simulink model "Cube"  (R2023a)
settings: Solver=FixedStepAuto  StartTime=0.0  StopTime=5  FixedStep=0.001  RelTol=1e-3
settings Model: Creator=Joseph Maher Labib  LastModifiedBy=totae
settings OptimizationCC: DefaultParameterBehavior=Inlined  EnhancedBackFolding=on  PassReuseOutputArgsAs=Individual arguments  ZeroExternalMemoryAtStartup=off  ZeroInternalMemoryAtStartup=off  OptimizeBlockOrder=speed  DifferentSizesBufferReuse=on  OptimizationCustomize=off  EfficientTunableParamExpr=on
settings DebuggingCC: ParameterTunabilityLossMsg=error
settings SFSimCC: MATLABDynamicMemAlloc=off
settings RTWCC: Description=Create Visual C/C++ Solution File for Embedded Coder  SystemTargetFile=ert.tlc  TemplateMakefile=RTW.MSVCBuild
settings CodeAppCC: ForceParamTrailComments=on  IgnoreCustomStorageClasses=off  OperatorAnnotations=on  SimulinkDataObjDesc=on  SFDataObjDesc=on  InsertBlockDesc=on
settings ERTTargetCC: TargetLangStandard=C99 (ISO)  GenerateSampleERTMain=on  SupportContinuousTime=on  InlinedParameterPlacement=NonHierarchical  ERTCustomFileTemplate=example_file_process.tlc

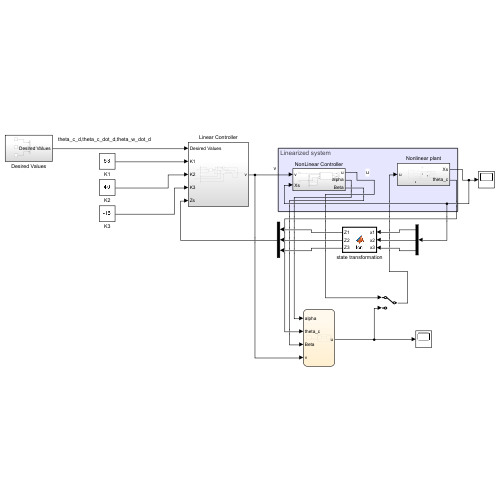
[thumbnail: Simulink's stored preview of the top-level diagram]
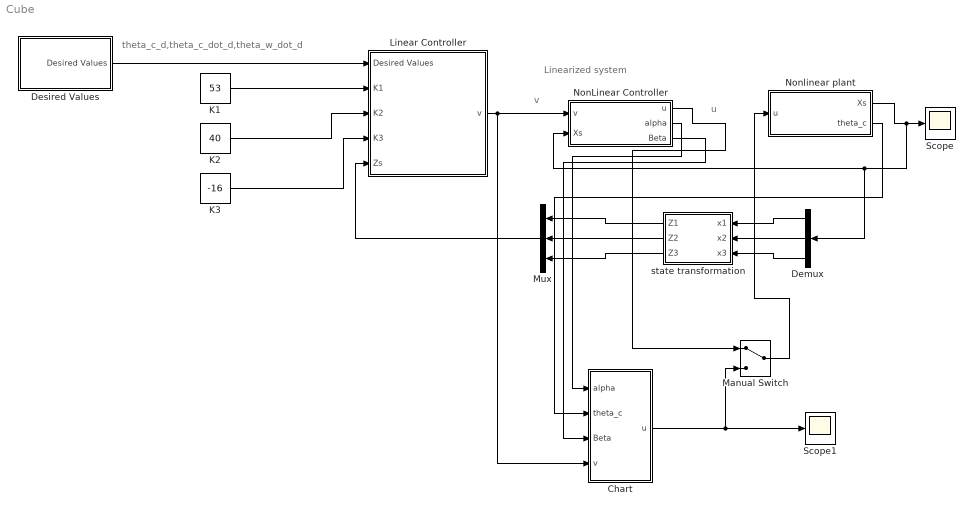
== system Cube ==
  note: Linearized system
  note: u
  note: v
  note: theta_c_d,theta_c_dot_d,theta_w_dot_d
  Chart : Stateflow chart  TreatAsAtomicUnit=on
  Demux : Demux  Outputs=3
  Desired Values : Subsystem
  K1 : Constant  Value=53
  K2 : Constant  Value=40
  K3 : Constant  Value=-16
  Linear Controller : Subsystem
  Manual Switch : ManualSwitch
  Mux : Mux  Inputs=3
  NonLinear Controller : Subsystem
  Nonlinear plant : Subsystem
  Scope : Scope
  Scope1 : Scope
  state transformation : MATLAB Function  TreatAsAtomicUnit=on
  wires:
  Desired Values/1(Desired Values) -> Linear Controller/1(Desired Values)
  Linear Controller/1(v) -> Chart/4(v), NonLinear Controller/1(v)
  NonLinear Controller/1(u) -> Manual Switch/1
  K1/1 -> Linear Controller/2(K1)
  K2/1 -> Linear Controller/3(K2)
  K3/1 -> Linear Controller/4(K3)
  Nonlinear plant/1(Xs) -> Demux/1, NonLinear Controller/2(Xs), Scope/1
  Demux/1 -> state transformation/1(x1)
  Demux/2 -> state transformation/2(x2)
  Demux/3 -> state transformation/3(x3)
  state transformation/2(Z2) -> Mux/2
  state transformation/1(Z1) -> Mux/1
  state transformation/3(Z3) -> Mux/3
  Mux/1 -> Linear Controller/5(Zs)
  NonLinear Controller/2(alpha) -> Chart/1(alpha)
  NonLinear Controller/3(Beta) -> Chart/3(Beta)
  Nonlinear plant/2(theta_c) -> Chart/2(theta_c)
  Chart/1(u) -> Manual Switch/2, Scope1/1
  Manual Switch/1 -> Nonlinear plant/1(u)

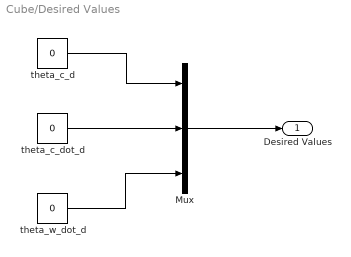
== system Cube/Desired Values ==
  Mux : Mux  Inputs=3
  theta_c_d : Constant  Value=0
  theta_c_dot_d : Constant  Value=0
  theta_w_dot_d : Constant  Value=0
  Desired Values : Outport
  wires:
  theta_c_dot_d/1 -> Mux/2
  theta_c_d/1 -> Mux/1
  theta_w_dot_d/1 -> Mux/3
  Mux/1 -> Desired Values/1

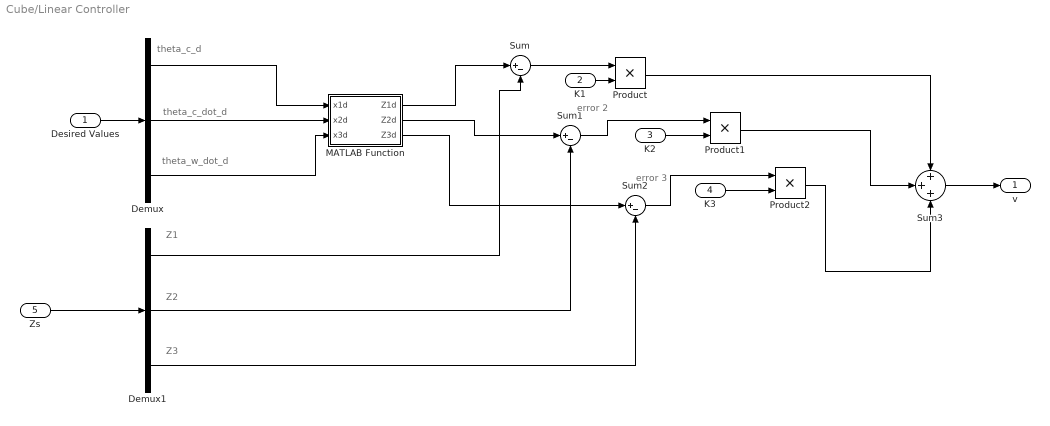
== system Cube/Linear Controller ==
  note: error 2
  note: error 3
  note: theta_w_dot_d
  note: theta_c_dot_d
  note: theta_c_d
  note: Z1
  note: Z2
  note: Z3
  Desired Values : Inport
  K1 : Inport  Port=2
  K2 : Inport  Port=3
  K3 : Inport  Port=4
  Zs : Inport  Port=5
  Demux : Demux  Outputs=3
  Demux1 : Demux  Outputs=3
  MATLAB Function : MATLAB Function  TreatAsAtomicUnit=on
  Product : Product
  Product1 : Product
  Product2 : Product
  Sum : Sum  Inputs=|+-
  Sum1 : Sum  Inputs=|+-
  Sum2 : Sum  Inputs=|+-
  Sum3 : Sum  Inputs=+++
  v : Outport
  wires:
  Desired Values/1 -> Demux/1
  Zs/1 -> Demux1/1
  Demux1/1 -> Sum/2
  Demux1/2 -> Sum1/2
  Demux1/3 -> Sum2/2
  K1/1 -> Product/2
  K2/1 -> Product1/2
  K3/1 -> Product2/2
  Product/1 -> Sum3/1
  Product1/1 -> Sum3/2
  Product2/1 -> Sum3/3
  Sum3/1 -> v/1
  Demux/1 -> MATLAB Function/1(x1d)
  Demux/2 -> MATLAB Function/2(x2d)
  Demux/3 -> MATLAB Function/3(x3d)
  MATLAB Function/1(Z1d) -> Sum/1
  MATLAB Function/3(Z3d) -> Sum2/1
  Sum2/1 -> Product2/1
  MATLAB Function/2(Z2d) -> Sum1/1
  Sum1/1 -> Product1/1
  Sum/1 -> Product/1

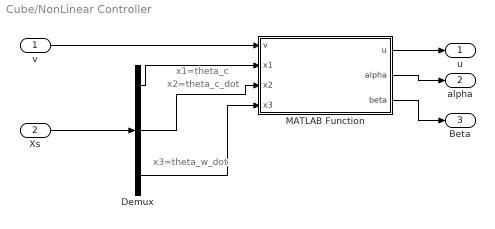
== system Cube/NonLinear Controller ==
  note: x1=theta_c
  note: x2=theta_c_dot
  note: x3=theta_w_dot
  v : Inport
  Xs : Inport  Port=2
  Demux : Demux  Outputs=3
  MATLAB Function : MATLAB Function  TreatAsAtomicUnit=on
  u : Outport
  alpha : Outport  Port=2
  Beta : Outport  Port=3
  wires:
  Xs/1 -> Demux/1
  v/1 -> MATLAB Function/1(v)
  Demux/1 -> MATLAB Function/2(x1)
  Demux/2 -> MATLAB Function/3(x2)
  Demux/3 -> MATLAB Function/4(x3)
  MATLAB Function/1(u) -> u/1
  MATLAB Function/2(alpha) -> alpha/1
  MATLAB Function/3(beta) -> Beta/1

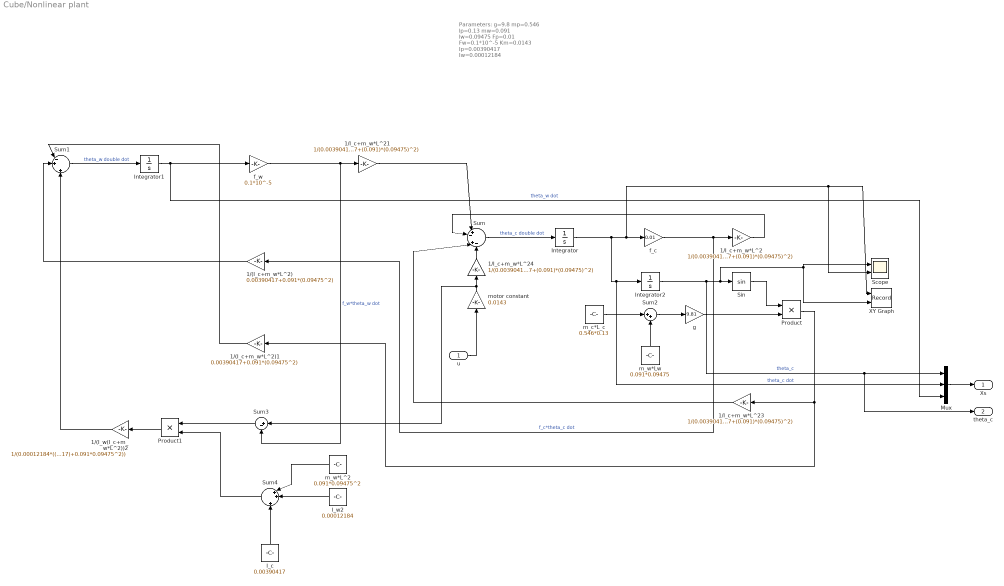
== system Cube/Nonlinear plant ==
  note: Parameters:
      | g=9.8
      | mp=0.546
      | lp=0.13
      | mw=0.091
      | lw=0.09475
      | Fp=0.01
      | Fw=0.1*10^-5
      | Km=0.0143
      | Ip=0.00390417
      | Iw=0.00012184
  u : Inport
  1/(I_c+m_w*L^2) : Gain  Gain=0.00390417+0.091*(0.09475^2)
  1/(I_c+m_w*L^2)1 : Gain  Gain=0.00390417+0.091*(0.09475^2)
  1/(I_w(I_c+m_w*L^2))2 : Gain  Gain=1/(0.00012184*((0.00390417)+0.091*0.09475^2))
  1/I_c+m_w*L^{2,21,23..24} (4 alike) : Gain  Gain=1/(0.00390417+(0.091)*(0.09475)^2)
  I_c : Constant  Value=0.00390417
  I_w2 : Constant  Value=0.00012184
  Integrator : Integrator
  Integrator1 : Integrator
  Integrator2 : Integrator
  Mux : Mux  Inputs=3
  Product : Product
  Product1 : Product
  Scope : Scope  NumInputPorts=2
  Sin : Trigonometry
  Sum : Sum  Inputs=|+-|+-
  Sum1 : Sum  Inputs=|-+|+
  Sum2 : Sum  Inputs=|++
  Sum3 : Sum  Inputs=|+-
  Sum4 : Sum  Inputs=|++|+
  XY Graph : Record  FileSettingsInternal="{\"entries\":[{\"content\":{\"excelSettings\":{\"content\":{},\"type\":\"Streamout.ExcelSettings\"}},\"type\":\"Streamout.FileSettingStorage\",\"uuid\":\"66a67cd6-09ae-4402-aca9-595720089f73\"}],\"packageUris\":[\"http://schema.mathworks.com/mf0/streamout_blocks/R2020a\"],\"version\":\"1.0\"}"  Layout=[1 1]  SignalsInternal="{\"entries\":[{\"content\":{\"signals\":[{\"content\":{\"blockPath\":[\"Cube/Nonlinear plant/XY Graph\"],\"dimensions\":[1],\"domain\":\"Cube/Nonlinear plant/XY Graph\",\"lineColor\":\"#0072bd\",\"plots\":[1],\"port\":1,\"signalID\":780,\"signalName\":\"theta_c dot\"},\"type\":\"RecordBlkView.Signal\",\"uuid\":\"a54ead99-843e-44f8-bb7c-9abc90be0651\"},{\"content\":{\"blockPath\":[\"Cube/Nonlinear plant/XY Graph\"],\"dimensions\":[1],\"domain\":\"Cube/Nonlinear plant/XY Graph\",\"lineColor\":\"#d95319\",\"plots\":[1],\"port\":2,\"signalID\":783,\"signalName\":\"theta_c\"},\"type\":\"RecordBlkView.Signal\",\"uuid\":\"b884fb43-d68a-49de-818e-e16d103745a3\"}]},\"type\":\"RecordBlkView.InputSignals\",\"uuid\":\"03c16a7e-bf53-4f70-b834-54f942da8cff\"}],\"packageUris\":[\"http://schema.mathworks.com/mf0/streamout_blocks/R2020a\"],\"version\":\"1.0\"}"  VisualizationBindings="{\"xyplotplugin\":{\"info\":[{\"series\":[{\"bindingParametersList\":[{\"parameter\":\"Y-Axis\",\"signalID\":780,\"signalName\":\"theta_c dot\"},{\"parameter\":\"X-Axis\",\"signalID\":783,\"signalName\":\"theta_c\"}],\"seriesID\":4721}],\"subplotID\":1}]}}"  CompatibilityTag=XY
  f_c : Gain  Gain=0.01
  f_w : Gain  Gain=0.1*10^-5
  g : Gain  Gain=9.81
  m_c*L_c : Constant  Value=0.546*0.13
  m_w*L^2 : Constant  Value=0.091*0.09475^2
  m_w*Lw : Constant  Value=0.091*0.09475
  motor constant : Gain  Gain=0.0143
  Xs : Outport
  theta_c : Outport  Port=2
  wires:
  I_w2/1 -> Sum4/2
  Integrator/1 -> Mux/2, Integrator2/1, XY Graph/1, Scope/2, f_c/1  "theta_c dot"
  Sin/1 -> Product/1
  I_c/1 -> Sum4/3
  Sum3/1 -> Product1/1
  1/I_c+m_w*L^21/1 -> Sum/1
  1/(I_w(I_c+m_w*L^2))2/1 -> Sum1/3
  Product1/1 -> 1/(I_w(I_c+m_w*L^2))2/1
  m_w*L^2/1 -> Sum4/1
  Integrator1/1 -> Mux/3, f_w/1  "theta_w dot"
  1/I_c+m_w*L^24/1 -> Sum/4
  m_w*Lw/1 -> Sum2/2
  1/(I_c+m_w*L^2)/1 -> Sum1/2
  Product/1 -> 1/(I_c+m_w*L^2)1/1, 1/I_c+m_w*L^23/1
  motor constant/1 -> Sum3/1, 1/I_c+m_w*L^24/1
  1/I_c+m_w*L^23/1 -> Sum/3
  Integrator2/1 -> theta_c/1, Mux/1, XY Graph/2, Scope/1, Sin/1  "theta_c"
  Sum4/1 -> Product1/2
  m_c*L_c/1 -> Sum2/1
  u/1 -> motor constant/1
  1/I_c+m_w*L^2/1 -> Sum/2
  Sum/1 -> Integrator/1  "theta_c double dot"
  f_w/1 -> 1/I_c+m_w*L^21/1, Sum3/2  "f_w*theta_w dot"
  f_c/1 -> 1/(I_c+m_w*L^2)/1, 1/I_c+m_w*L^2/1  "f_c*theta_c dot"
  g/1 -> Product/2
  Sum2/1 -> g/1
  Sum1/1 -> Integrator1/1  "theta_w double dot"
  1/(I_c+m_w*L^2)1/1 -> Sum1/1
  Mux/1 -> Xs/1

== stateflow chart Cube/Chart ==
  state On
    state Balanced
      entry:
      during:
      u=0;
    state Falling
      entry:
      during:
      u=alpha+Beta*v;
    (default) -> Balanced
    Balanced -> Falling : [theta_c >5 || theta_c<-5]
    Falling -> Balanced : [theta_c>-5 && theta_c<5]
  state Off
    entry:
    during:
    u=0;
  (default) -> Off
  On -> Off : [button_pressed==0]
  Off -> On : [button_pressed==1]
  data: alpha input; theta_c input; Beta input; v input; u output double; button_pressed local double

== matlab function Cube/NonLinear Controller/MATLAB Function ==
  data: v input; u output; x1 input; x2 input; x3 input; alpha output; beta output
function [u,alpha,beta] = fcn(v,x1,x2,x3)

%Parameters: 
g=9.8;
mp=0.546;
lp=0.13;
mw=0.091;
lw=0.09475;
Fp=0.01;
Fw=0.1*10^-5;
Km=0.0143;
Ip=0.00390417;
Iw=0.00012184;

alpha =(x2*((49*g*x2*sin(x1)*(lp*mp + lw*mw))/(60*(mw*lw^2 + Ip)) - (g*cos(x1)*((11*Fw)/(60*(mw*lw^2 + Ip)) - Fw/(Iw*(mw*lw^2 + Ip)))*(lp*mp + lw*mw))/(mw*lw^2 + Ip) + (g*cos(x1)*((49*Fp)/(60*(mw*lw^2 + Ip)) - 467/225)*(lp*mp + lw*mw))/(mw*lw^2 + Ip)) + ((Fp*x2 - g*sin(x1)*(lp*mp + lw*mw))/(mw*lw^2 + Ip) + (mw*lw^2 + Ip + Iw - Fw*x3)/(Iw*(mw*lw^2 + Ip)))*((Fw*((49*Fp)/(60*(mw*lw^2 + Ip)) - 467/225))/(mw*lw^2 + Ip) - (Fw*((11*Fw)/(60*(mw*lw^2 + Ip)) - Fw/(Iw*(mw*lw^2 + Ip))))/(Iw*(mw*lw^2 + Ip))) - ((Fw*x3 - Fp*x2 + g*sin(x1)*(lp*mp + lw*mw))*((Fp*((49*Fp)/(60*(mw*lw^2 + Ip)) - 467/225))/(mw*lw^2 + Ip) - (Fp*((11*Fw)/(60*(mw*lw^2 + Ip)) - Fw/(Iw*(mw*lw^2 + Ip))))/(mw*lw^2 + Ip) + (49*g*cos(x1)*(lp*mp + lw*mw))/(60*(mw*lw^2 + Ip))))/(mw*lw^2 + Ip))/((Km*((Fp*((49*Fp)/(60*(mw*lw^2 + Ip)) - 467/225))/(mw*lw^2 + Ip) - (Fp*((11*Fw)/(60*(mw*lw^2 + Ip)) - Fw/(Iw*(mw*lw^2 + Ip))))/(mw*lw^2 + Ip) + (49*g*cos(x1)*(lp*mp + lw*mw))/(60*(mw*lw^2 + Ip))))/(mw*lw^2 + Ip) + (Km*(mw*lw^2 + Ip)*((Fw*((49*Fp)/(60*(mw*lw^2 + Ip)) - 467/225))/(mw*lw^2 + Ip) - (Fw*((11*Fw)/(60*(mw*lw^2 + Ip)) - Fw/(Iw*(mw*lw^2 + Ip))))/(Iw*(mw*lw^2 + Ip))))/Iw);
 
beta =1/((Km*((Fp*((49*Fp)/(60*(mw*lw^2 + Ip)) - 467/225))/(mw*lw^2 + Ip) - (Fp*((11*Fw)/(60*(mw*lw^2 + Ip)) - Fw/(Iw*(mw*lw^2 + Ip))))/(mw*lw^2 + Ip) + (49*g*cos(x1)*(lp*mp + lw*mw))/(60*(mw*lw^2 + Ip))))/(mw*lw^2 + Ip) + (Km*(mw*lw^2 + Ip)*((Fw*((49*Fp)/(60*(mw*lw^2 + Ip)) - 467/225))/(mw*lw^2 + Ip) - (Fw*((11*Fw)/(60*(mw*lw^2 + Ip)) - Fw/(Iw*(mw*lw^2 + Ip))))/(Iw*(mw*lw^2 + Ip))))/Iw);


u=alpha+beta*v

== matlab function Cube/state transformation ==
  data: x1 input; Z1 output; x2 input; x3 input; Z2 output; Z3 output
function [Z1,Z2,Z3] = fcn(x1,x2,x3)

%Parameters 
g=9.8;
mp=0.546;
lp=0.13;
mw=0.091;
lw=0.09475;
Fp=0.01;
Fw=0.1*10^-5;
Km=0.0143;
Ip=0.00390417;
Iw=0.00012184;


Z1 = (-467/225)*x1+(11/60)*x2+x3;
Z2 =(Fp*x2 - g*sin(x1)*(lp*mp + lw*mw))/(mw*lw^2 + Ip) - (467*x2)/225 + (11*(Fw*x3 - Fp*x2+ g*sin(x1)*(lp*mp + lw*mw)))/(60*(mw*lw^2 + Ip)) + (mw*lw^2 + Ip + Iw - Fw*x3)/(Iw*(mw*lw^2 + Ip));
Z3 =((11*Fw)/(60*(mw*lw^2 + Ip)) - Fw/(Iw*(mw*lw^2 + Ip)))*((Fp*x2 - g*sin(x1)*(lp*mp + lw*mw))/(mw*lw^2 + Ip) + (mw*lw^2 + Ip + Iw - Fw*x3)/(Iw*(mw*lw^2 + Ip))) + (((49*Fp)/(60*(mw*lw^2 + Ip)) - 467/225)*(Fw*x3 - Fp*x2 + g*sin(x1)*(lp*mp + lw*mw)))/(mw*lw^2 + Ip) - (49*g*x2*cos(x1)*(lp*mp + lw*mw))/(60*(mw*lw^2 + Ip));

== matlab function Cube/Linear Controller/MATLAB Function ==
  data: x1d input; Z1d output; x2d input; x3d input; Z2d output; Z3d output
function [Z1d,Z2d,Z3d] = fcn(x1d,x2d,x3d)

%Parameters 
g=9.8
mp=0.546
lp=0.13
mw=0.091
lw=0.09475
Fp=0.01
Fw=0.1*10^-5
Km=0.0143
Ip=0.00390417
Iw=0.00012184

Z1d = (-467/225)*x1d+(11/60)*x2d+x3d;
Z2d= (Fp*x2d - g*sin(x1d)*(lp*mp + lw*mw))/(mw*lw^2 + Ip) - (467*x2d)/225 + (11*(Fw*x3d - Fp*x2d+ g*sin(x1d)*(lp*mp + lw*mw)))/(60*(mw*lw^2 + Ip)) + (mw*lw^2 + Ip + Iw - Fw*x3d)/(Iw*(mw*lw^2 + Ip));
Z3d=(11*Fw)/(60*(mw*lw^2 + Ip)) - Fw/(Iw*(mw*lw^2 + Ip))*((Fp*x2d - g*sin(x1d)*(lp*mp + lw*mw))/(mw*lw^2 + Ip) + (mw*lw^2 + Ip + Iw - Fw*x3d)/(Iw*(mw*lw^2 + Ip))) + (((49*Fp)/(60*(mw*lw^2 + Ip)) - 467/225)*(Fw*x3d - Fp*x2d + g*sin(x1d)*(lp*mp + lw*mw)))/(mw*lw^2 + Ip) - (49*g*x2d*cos(x1d)*(lp*mp + lw*mw))/(60*(mw*lw^2 + Ip));
